simulink model "LQR_2_QuadrotorModel"  (R2023b)
settings: Solver=VariableStepAuto  StartTime=0.0  StopTime=time_model  RelTol=1e-3
values from neighbouring files (symbols this model uses):
  A_flap = [c_a, c_b, 0 ... (first row only)    [LQR_calculate.m]    (also in LQR_feedback.m; LQR_linearized_test.m; MPC_test.m; MPC_test_1.m)
  A_ind = [c_d, 0, 0 ... (first row only)    [LQR_calculate.m]    (also in LQR_feedback.m; LQR_linearized_test.m; MPC_test.m; MPC_test_1.m)
  C_drag = 0    [LQR_calculate.m]    (also in LQR_feedback.m = C_drag_arr(i); LQR_linearized_test.m = C_drag_arr(i); MPC_test.m = C_drag_arr(i); MPC_test_1.m = C_drag_arr(i))
  demp = 0    [LQR_feedback.m]    (also in LQR_linearized_test.m; MPC_params.m; MPC_test_1.m; initQuadrotorData.m)
  forward_1 = 20    [LQR_feedback.m]    (also in LQR_linearized_test.m; MPC_test_1.m)
  forward_2 = 20    [LQR_feedback.m]    (also in LQR_linearized_test.m; MPC_test_1.m)
  g = 9.81    [LQR_calculate.m]    (also in LQR_feedback.m = 9.8; LQR_linearized_test.m = 9.8; LQR_testing_gpt.m; MPC_params.m = 9.8)
  Ix = m/3*a^2/12+2*0.045*l^2    (= 0.00211347222222)    [LQR_calculate.m]    (also in LQR_feedback.m; LQR_linearized_test.m; LQR_testing_gpt.m = 0.0081; MPC_params.m)
  Iy = m/3*a^2/12+4*0.045*l^2    (= 0.00413847222222)    [LQR_calculate.m]    (also in LQR_feedback.m = 0.00211347222222; LQR_linearized_test.m = 0.00211347222222; LQR_testing_gpt.m = 0.0081; MPC_params.m = 0.00211347222222)
  Iz = m/3*a^2/4+2*0.045*l^2    (= 0.00229041666667)    [LQR_calculate.m]    (also in LQR_feedback.m = 0.00431541666667; LQR_linearized_test.m = 0.00431541666667; LQR_testing_gpt.m = 0.0142; MPC_params.m = 0.00431541666667)
  J = 2.5*10^(-6)    (= 2.5e-06)    [LQR_calculate.m]    (also in LQR_feedback.m; LQR_linearized_test.m; MPC_params.m; MPC_test.m)
  K = Y * inv(P)    [LQR_calculate.m]    (also in LQR_feedback.m = [Kx;Ky;Kz;Kphi;Ktheta;-Kpsi])
  Ke = ke    (= 0.0073)    [LQR_calculate.m]    (also in LQR_feedback.m = 0.00734; LQR_linearized_test.m = 0.00734; MPC_params.m = 0.00734; MPC_test.m)
  kf = ks*r^2*airDensity*Sblade/2    (= 1.57565625e-05)    [LQR_calculate.m]    (also in LQR_feedback.m; LQR_linearized_test.m; MPC_params.m; MPC_test.m)
  Km = kt    (= 0.0073)    [LQR_calculate.m]    (also in LQR_feedback.m = 0.00734; LQR_linearized_test.m = 0.00734; MPC_params.m = 0.00734; MPC_test.m)
  kv = 1300    [LQR_feedback.m]    (also in LQR_linearized_test.m; MPC_test_1.m; initQuadrotorData.m)
  L = La    (= 5e-05)    [LQR_calculate.m]    (also in LQR_feedback.m = 0.0001; LQR_linearized_test.m = 0.0001; MPC_params.m = 0.0001; MPC_test.m)
  l = 0.15    [LQR_calculate.m]    (also in LQR_feedback.m; LQR_linearized_test.m; MPC_params.m; MPC_test.m)
  m = size(B, 2)    [LQR_calculate.m]    (also in LQR_feedback.m = 0.65; LQR_linearized_test.m = 0.65; LQR_testing_gpt.m = 1; MPC_params.m = 0.65)
  maxU = 16    [LQR_calculate.m]    (also in LQR_feedback.m; LQR_linearized_test.m; MPC_params.m; MPC_test.m = 11)
  Mode = 3    [LQR_feedback.m]    (also in LQR_linearized_test.m; MPC_test_1.m = 1)
  phi0 = 0    [LQR_feedback.m]    (also in LQR_linearized_test.m; MPC_test_1.m)
  psi0 = pi/2    (= 1.57079632679)    [LQR_feedback.m]    (also in LQR_linearized_test.m; MPC_test_1.m = 0)
  R = eye(4)    [LQR_calculate.m]    (also in LQR_feedback.m = 0.058; LQR_linearized_test.m = 0.058; LQR_testing_gpt.m = diag([0.1, 10, 100, 10]); MPC_params.m = 0.058)
  rho = 1.225    [LQR_calculate.m]    (also in LQR_feedback.m; LQR_linearized_test.m; MPC_params.m; MPC_test.m)
  S = l*c*4+a*b    (= 0.0169)    [LQR_calculate.m]    (also in LQR_feedback.m; LQR_linearized_test.m; MPC_params.m; MPC_test.m)
  theta0 = 0    [LQR_feedback.m]    (also in LQR_linearized_test.m; MPC_test_1.m)
  total_time = 60    [LQR_feedback.m]    (also in LQR_linearized_test.m; MPC_test_1.m)
  up_down = 5    [LQR_feedback.m]    (also in LQR_linearized_test.m; MPC_test_1.m)
  x0 = 0    [LQR_feedback.m]    (also in LQR_linearized_test.m; MPC_test_1.m; init_nmpc.m = zeros(nx,1))
  y0 = 0    [LQR_feedback.m]    (also in LQR_linearized_test.m; MPC_test_1.m)
  z0 = 0    [LQR_feedback.m]    (also in LQR_linearized_test.m; MPC_test_1.m)
libraries: sharedtransform x1
settings Model: Creator=Degra  LastModifiedBy=Degra

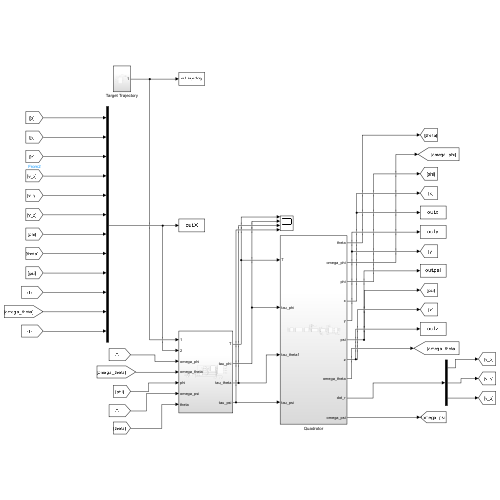
[thumbnail: Simulink's stored preview of the top-level diagram]
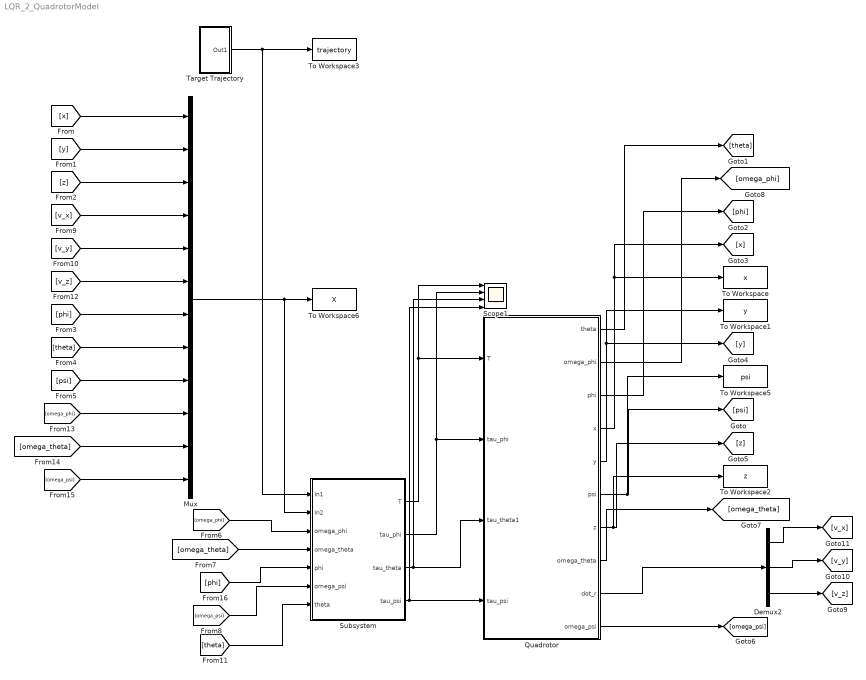
== system LQR_2_QuadrotorModel ==
  Demux2 : Demux  Outputs=3
  Mux : Mux  Inputs=12
  Quadrotor : Subsystem
  Scope1 : Scope  NumInputPorts=4
  Subsystem : Subsystem
  Target Trajectory : Subsystem
  To Workspace : ToWorkspace  VariableName=x  SaveFormat=Timeseries  SampleTime=-1
  To Workspace1 : ToWorkspace  VariableName=y  SaveFormat=Timeseries  SampleTime=-1
  To Workspace2 : ToWorkspace  VariableName=z  SaveFormat=Timeseries  SampleTime=-1
  To Workspace3 : ToWorkspace  VariableName=trajectory  SaveFormat=Timeseries  SampleTime=-1
  To Workspace5 : ToWorkspace  VariableName=psi  SaveFormat=Timeseries  SampleTime=-1
  To Workspace6 : ToWorkspace  VariableName=X  SaveFormat=Timeseries  SampleTime=-1
  wires:
  [x] -> Mux/1
  Demux2/3 -> [v_z]
  Demux2/2 -> [v_y]
  [phi] -> Subsystem/5(phi)
  [omega_psi] -> Mux/12
  [y] -> Mux/2
  [z] -> Mux/3
  [phi] -> Mux/7
  [theta] -> Subsystem/7(theta)
  [v_y] -> Mux/5
  [omega_psi] -> Subsystem/6(omega_psi)
  [v_x] -> Mux/4
  Demux2/1 -> [v_x]
  Quadrotor/5(y) -> To Workspace1/1, [y]
  Quadrotor/4(x) -> [x], To Workspace/1
  [omega_theta] -> Mux/11
  [v_z] -> Mux/6
  [psi] -> Mux/9
  [theta] -> Mux/8
  [omega_phi] -> Mux/10
  Target Trajectory/1(Out1) -> To Workspace3/1, Subsystem/1(In1)
  Mux/1 -> Subsystem/2(In2), To Workspace6/1
  Quadrotor/10(omega_psi) -> [omega_psi]
  Quadrotor/9(dot_r) -> Demux2/1
  [omega_theta] -> Subsystem/4(omega_theta)
  [omega_phi] -> Subsystem/3(omega_phi)
  Subsystem/4(tau_psi) -> Scope1/4, Quadrotor/4(tau_psi)
  Subsystem/3(tau_theta) -> Quadrotor/3(tau_theta1), Scope1/3
  Subsystem/2(tau_phi) -> Quadrotor/2(tau_phi), Scope1/2
  Subsystem/1(T) -> Scope1/1, Quadrotor/1(T)
  Quadrotor/3(phi) -> [phi]
  Quadrotor/2(omega_phi) -> [omega_phi]
  Quadrotor/1(theta) -> [theta]
  Quadrotor/8(omega_theta) -> [omega_theta]
  Quadrotor/7(z) -> To Workspace2/1, [z]
  Quadrotor/6(psi) -> [psi], To Workspace5/1

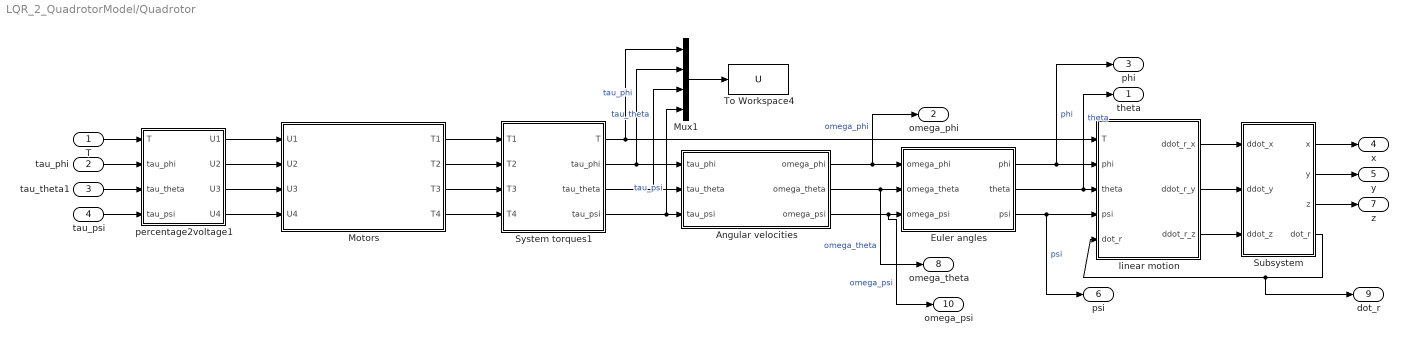
== system LQR_2_QuadrotorModel/Quadrotor ==
  T : Inport
  tau_phi : Inport  Port=2
  tau_theta1 : Inport  Port=3
  tau_psi : Inport  Port=4
  Angular velocities : Subsystem
  Euler angles : Subsystem
  Motors : Subsystem
  Mux1 : Mux
  Subsystem : Subsystem
  System torques1 : Subsystem
  To Workspace4 : ToWorkspace  VariableName=U  SaveFormat=Timeseries  SampleTime=-1
  linear motion : Subsystem
  percentage2voltage1 : Subsystem
  theta : Outport
  omega_phi : Outport  Port=2
  phi : Outport  Port=3
  x : Outport  Port=4
  y : Outport  Port=5
  psi : Outport  Port=6
  z : Outport  Port=7
  omega_theta : Outport  Port=8
  dot_r : Outport  Port=9
  omega_psi : Outport  Port=10
  wires:
  Angular velocities/1(omega_phi) -> Euler angles/1(omega_phi), omega_phi/1  "omega_phi"
  linear motion/2(ddot_r_y) -> Subsystem/2(ddot_y)
  Subsystem/4(dot_r) -> linear motion/5(dot_r), dot_r/1
  Angular velocities/2(omega_theta) -> Euler angles/2(omega_theta), omega_theta/1  "omega_theta"
  percentage2voltage1/4(U4) -> Motors/4(U4)
  tau_psi/1 -> percentage2voltage1/4(tau_psi)
  Euler angles/1(phi) -> linear motion/2(phi), phi/1  "phi"
  Euler angles/2(theta) -> linear motion/3(theta), theta/1  "theta"
  T/1 -> percentage2voltage1/1(T)
  System torques1/3(tau_theta) -> Mux1/3, Angular velocities/2(tau_theta)  "tau_theta"
  linear motion/3(ddot_r_z) -> Subsystem/3(ddot_z)
  linear motion/1(ddot_r_x) -> Subsystem/1(ddot_x)
  Motors/3(T3) -> System torques1/3(T3)
  tau_phi/1 -> percentage2voltage1/2(tau_phi)
  Euler angles/3(psi) -> linear motion/4(psi), psi/1  "psi"
  tau_theta1/1 -> percentage2voltage1/3(tau_theta)
  Motors/2(T2) -> System torques1/2(T2)
  Subsystem/3(z) -> z/1
  Motors/1(T1) -> System torques1/1(T1)
  Subsystem/1(x) -> x/1
  Motors/4(T4) -> System torques1/4(T4)
  Angular velocities/3(omega_psi) -> omega_psi/1, Euler angles/3(omega_psi)  "omega_psi"
  percentage2voltage1/3(U3) -> Motors/3(U3)
  percentage2voltage1/2(U2) -> Motors/2(U2)
  percentage2voltage1/1(U1) -> Motors/1(U1)
  System torques1/2(tau_phi) -> Mux1/2, Angular velocities/1(tau_phi)  "tau_phi"
  Subsystem/2(y) -> y/1
  System torques1/4(tau_psi) -> Mux1/4, Angular velocities/3(tau_psi)  "tau_psi"
  Mux1/1 -> To Workspace4/1
  System torques1/1(T) -> Mux1/1, linear motion/1(T)

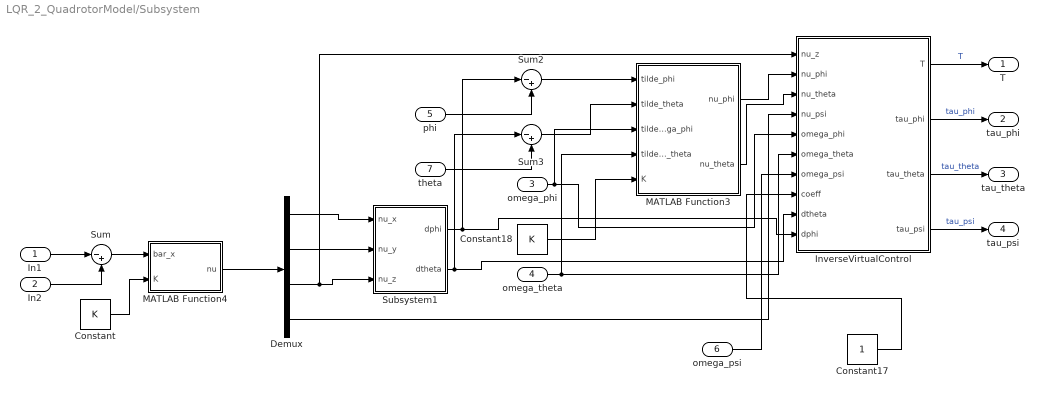
== system LQR_2_QuadrotorModel/Subsystem ==
  In1 : Inport
  In2 : Inport  Port=2
  omega_phi : Inport  Port=3
  omega_theta : Inport  Port=4
  phi : Inport  Port=5
  omega_psi : Inport  Port=6
  theta : Inport  Port=7
  Constant : Constant  Value=K
  Constant17 : Constant
  Constant18 : Constant  Value=K
  Demux : Demux
  InverseVirtualControl : Subsystem
  MATLAB Function3 : MATLAB Function  TreatAsAtomicUnit=on
  MATLAB Function4 : MATLAB Function  TreatAsAtomicUnit=on
  Subsystem1 : Subsystem
  Sum : Sum  Inputs=|-+
  Sum2 : Sum  Inputs=|-+
  Sum3 : Sum  Inputs=|-+
  T : Outport
  tau_phi : Outport  Port=2
  tau_theta : Outport  Port=3
  tau_psi : Outport  Port=4
  wires:
  In1/1 -> Sum/1
  Demux/1 -> Subsystem1/1(nu_x)
  omega_phi/1 -> InverseVirtualControl/5(omega_phi), MATLAB Function3/3(tilde_omega_phi)
  In2/1 -> Sum/2
  MATLAB Function4/1(nu) -> Demux/1
  Sum/1 -> MATLAB Function4/1(bar_x)
  Constant/1 -> MATLAB Function4/2(K)
  Demux/2 -> Subsystem1/2(nu_y)
  Subsystem1/2(dtheta) -> Sum3/1, InverseVirtualControl/9(dtheta)
  Demux/4 -> InverseVirtualControl/4(nu_psi)
  Demux/3 -> InverseVirtualControl/1(nu_z), Subsystem1/3(nu_z)
  omega_theta/1 -> InverseVirtualControl/6(omega_theta), MATLAB Function3/4(tilde_omega_theta)
  Sum2/1 -> MATLAB Function3/1(tilde_phi)
  phi/1 -> Sum2/2
  omega_psi/1 -> InverseVirtualControl/7(omega_psi)
  theta/1 -> Sum3/2
  Subsystem1/1(dphi) -> InverseVirtualControl/10(dphi), Sum2/1
  Sum3/1 -> MATLAB Function3/2(tilde_theta)
  Constant17/1 -> InverseVirtualControl/8(coeff)
  Constant18/1 -> MATLAB Function3/5(K)
  MATLAB Function3/2(nu_theta) -> InverseVirtualControl/3(nu_theta)
  MATLAB Function3/1(nu_phi) -> InverseVirtualControl/2(nu_phi)
  InverseVirtualControl/2(tau_phi) -> tau_phi/1  "tau_phi"
  InverseVirtualControl/1(T) -> T/1  "T"
  InverseVirtualControl/4(tau_psi) -> tau_psi/1  "tau_psi"
  InverseVirtualControl/3(tau_theta) -> tau_theta/1  "tau_theta"

== system LQR_2_QuadrotorModel/Target Trajectory ==
  Clock : Clock
  Clock2 : Clock
  Constant1 : Constant  Value=Mode
  Constant13 : Constant  Value=forward_2
  Constant14 : Constant  Value=total_time
  Constant15 : Constant  Value=up_down
  Constant16 : Constant  Value=forward_1
  MATLAB Function : MATLAB Function  TreatAsAtomicUnit=on
  MATLAB Function1 : MATLAB Function  TreatAsAtomicUnit=on
  Multiport Switch : MultiPortSwitch  Inputs=2  SaturateOnIntegerOverflow=off  InputSameDT=off
  Out1 : Outport
  wires:
  Constant1/1 -> Multiport Switch/1
  Clock/1 -> MATLAB Function1/1(t)
  Constant13/1 -> MATLAB Function/2(forward_20)
  Clock2/1 -> MATLAB Function/1(t)
  MATLAB Function/1(x_ref) -> Multiport Switch/3
  Constant14/1 -> MATLAB Function/5(total_time)
  Multiport Switch/1 -> Out1/1
  Constant16/1 -> MATLAB Function/3(forward_10)
  MATLAB Function1/1(x_ref) -> Multiport Switch/2
  Constant15/1 -> MATLAB Function/4(up_down)

== system LQR_2_QuadrotorModel/Quadrotor/Angular velocities ==
  tau_phi : Inport
  tau_theta : Inport  Port=2
  tau_psi : Inport  Port=3
  Subsystem1 : Subsystem
  Subsystem2 : Subsystem
  Subsystem3 : Subsystem
  omega_phi : Outport
  omega_theta : Outport  Port=2
  omega_psi : Outport  Port=3
  wires:
  Subsystem2/1(omega_theta) -> omega_theta/1, Subsystem1/2(omega_theta), Subsystem3/3(omega_theta)  "omega_theta"
  tau_theta/1 -> Subsystem2/1(tau_theta)
  Subsystem1/1(omega_phi) -> omega_phi/1, Subsystem3/2(omega_phi), Subsystem2/2(omega_phi)  "omega_phi"
  Subsystem3/1(omega_psi) -> omega_psi/1, Subsystem2/3(omega_psi), Subsystem1/3(omega_psi)  "omega_psi"
  tau_phi/1 -> Subsystem1/1(tau_phi)
  tau_psi/1 -> Subsystem3/1(tau_psi)

== system LQR_2_QuadrotorModel/Quadrotor/Euler angles ==
  omega_phi : Inport
  omega_theta : Inport  Port=2
  omega_psi : Inport  Port=3
  Subsystem1 : Subsystem
  Subsystem2 : Subsystem
  Subsystem3 : Subsystem
  phi : Outport
  theta : Outport  Port=2
  psi : Outport  Port=3
  wires:
  Subsystem2/1(theta) -> theta/1, Subsystem1/2(theta), Subsystem3/4(theta)  "theta"
  Subsystem1/1(phi) -> phi/1, Subsystem3/1(phi), Subsystem2/1(phi)  "phi"
  omega_theta/1 -> Subsystem3/2(omega_theta), Subsystem1/3(omega_theta), Subsystem2/2(omega_theta)
  omega_psi/1 -> Subsystem2/3(omega_psi), Subsystem3/3(omega_psi), Subsystem1/4(omega_psi)
  omega_phi/1 -> Subsystem1/1(omega_phi)
  Subsystem3/1(psi) -> psi/1  "psi"

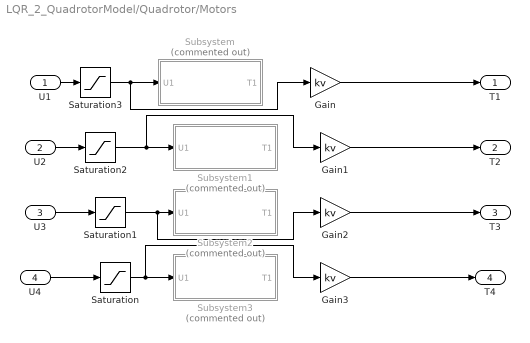
== system LQR_2_QuadrotorModel/Quadrotor/Motors ==
  U1 : Inport
  U2 : Inport  Port=2
  U3 : Inport  Port=3
  U4 : Inport  Port=4
  Gain{,1..3} (4 alike) : Gain  Gain=kv
  Saturation{,1..3} (4 alike) : Saturate  UpperLimit=maxU  LowerLimit=-maxU
  Subsystem : Subsystem  Commented=on
  Subsystem1 : Subsystem  Commented=on
  Subsystem2 : Subsystem  Commented=on
  Subsystem3 : Subsystem  Commented=on
  T1 : Outport
  T2 : Outport  Port=2
  T3 : Outport  Port=3
  T4 : Outport  Port=4
  wires:
  U4/1 -> Saturation/1
  U1/1 -> Saturation3/1
  U3/1 -> Saturation1/1
  U2/1 -> Saturation2/1
  Gain/1 -> T1/1
  Gain1/1 -> T2/1
  Gain2/1 -> T3/1
  Gain3/1 -> T4/1
  Saturation/1 -> Gain3/1, Subsystem3/1(U1)
  Saturation1/1 -> Gain2/1, Subsystem2/1(U1)
  Saturation2/1 -> Gain1/1, Subsystem1/1(U1)
  Saturation3/1 -> Gain/1, Subsystem/1(U1)

== system LQR_2_QuadrotorModel/Quadrotor/Subsystem ==
  ddot_x : Inport
  ddot_y : Inport  Port=2
  ddot_z : Inport  Port=3
  Integrator10 : Integrator  InitialCondition=z0
  Integrator11 : Integrator
  Integrator6 : Integrator  InitialCondition=x0
  Integrator7 : Integrator
  Integrator8 : Integrator  InitialCondition=y0
  Integrator9 : Integrator
  Mux : Mux  Inputs=3
  x : Outport
  y : Outport  Port=2
  z : Outport  Port=3
  dot_r : Outport  Port=4
  wires:
  Integrator9/1 -> Mux/2, Integrator8/1
  Integrator7/1 -> Mux/1, Integrator6/1
  Integrator10/1 -> z/1  "z"
  Integrator11/1 -> Mux/3, Integrator10/1
  Integrator8/1 -> y/1  "y"
  ddot_x/1 -> Integrator7/1
  Mux/1 -> dot_r/1  "dot_r"
  Integrator6/1 -> x/1  "x"
  ddot_y/1 -> Integrator9/1
  ddot_z/1 -> Integrator11/1

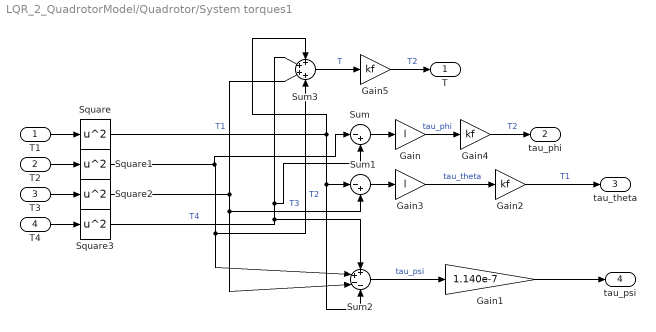
== system LQR_2_QuadrotorModel/Quadrotor/System torques1 ==
  T1 : Inport
  T2 : Inport  Port=2
  T3 : Inport  Port=3
  T4 : Inport  Port=4
  Gain : Gain  Gain=l
  Gain1 : Gain  Gain=1.140e-7
  Gain2 : Gain  Gain=kf
  Gain3 : Gain  Gain=l
  Gain4 : Gain  Gain=kf
  Gain5 : Gain  Gain=kf
  Square{,1..3} (4 alike) : Math  Operator=square
  Sum : Sum  Inputs=|-+
  Sum1 : Sum  Inputs=|-+
  Sum2 : Sum  Inputs=++--
  Sum3 : Sum  Inputs=++++
  T : Outport
  tau_phi : Outport  Port=2
  tau_theta : Outport  Port=3
  tau_psi : Outport  Port=4
  wires:
  T3/1 -> Square2/1
  T4/1 -> Square3/1
  Sum2/1 -> Gain1/1  "tau_psi"
  T1/1 -> Square/1
  Sum/1 -> Gain/1
  Sum1/1 -> Gain3/1
  Sum3/1 -> Gain5/1  "T"
  T2/1 -> Square1/1
  Gain3/1 -> Gain2/1  "tau_theta"
  Gain/1 -> Gain4/1  "tau_phi"
  Gain1/1 -> tau_psi/1
  Square/1 -> Sum1/1, Sum2/4, Sum3/1  "T1"
  Square1/1 -> Sum/1, Sum2/2, Sum3/4  "T2"
  Square2/1 -> Sum1/2, Sum2/3, Sum3/3  "T3"
  Square3/1 -> Sum/2, Sum3/2, Sum2/1  "T4"
  Gain4/1 -> tau_phi/1  "T2"
  Gain2/1 -> tau_theta/1  "T1"
  Gain5/1 -> T/1  "T2"

== system LQR_2_QuadrotorModel/Quadrotor/linear motion ==
  T : Inport
  phi : Inport  Port=2
  theta : Inport  Port=3
  psi : Inport  Port=4
  dot_r : Inport  Port=5
  Subsystem : Subsystem
  Subsystem1 : Subsystem
  Subsystem2 : Subsystem
  Subsystem3 : Subsystem
  ddot_r_x : Outport
  ddot_r_y : Outport  Port=2
  ddot_r_z : Outport  Port=3
  wires:
  T/1 -> Subsystem/1(T), Subsystem2/2(T), Subsystem3/1(T), Subsystem1/1(T)
  theta/1 -> Subsystem/2(theta), Subsystem2/3(theta), Subsystem3/4(theta), Subsystem1/3(theta)
  phi/1 -> Subsystem/3(phi), Subsystem2/4(phi), Subsystem3/2(phi), Subsystem1/2(phi)
  Subsystem1/3((F_ind+F_flap+F_drag)_z) -> Subsystem/4((F_ind+F_flap+F_drag)_z)
  psi/1 -> Subsystem3/5(psi), Subsystem2/1(psi), Subsystem1/4(psi)
  dot_r/1 -> Subsystem1/5(dot_r)
  Subsystem1/2((F_ind+F_flap+F_drag)_y) -> Subsystem2/5((F_ind+F_flap+F_drag)_y)
  Subsystem1/1((F_ind+F_flap+F_drag)_x) -> Subsystem3/3((F_ind+F_flap+F_drag)_x)
  Subsystem3/1(ddot_r_x) -> ddot_r_x/1  "ddot_r_x"
  Subsystem2/1(ddot_r_y) -> ddot_r_y/1  "ddot_r_y"
  Subsystem/1(ddot_r_z) -> ddot_r_z/1  "ddot_r_z"

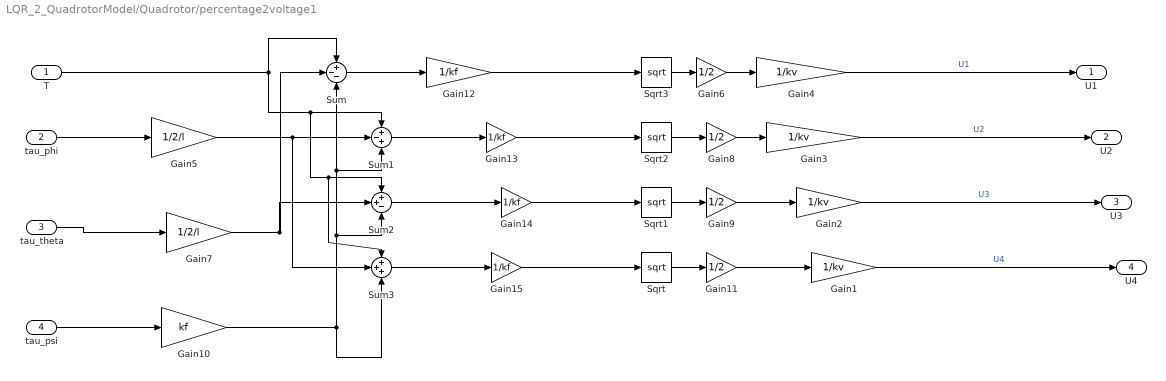
== system LQR_2_QuadrotorModel/Quadrotor/percentage2voltage1 ==
  T : Inport
  tau_phi : Inport  Port=2
  tau_theta : Inport  Port=3
  tau_psi : Inport  Port=4
  Gain{1..4} (4 alike) : Gain  Gain=1/kv
  Gain10 : Gain  Gain=kf
  Gain{6,8..9,11} (4 alike) : Gain  Gain=1/2
  Gain{12..15} (4 alike) : Gain  Gain=1/kf
  Gain5 : Gain  Gain=1/2/l
  Gain7 : Gain  Gain=1/2/l
  Sqrt{,1..3} (4 alike) : Sqrt
  Sum : Sum  Inputs=+--
  Sum1 : Sum  Inputs=+-+
  Sum2 : Sum  Inputs=++-
  Sum3 : Sum  Inputs=+++
  U1 : Outport
  U2 : Outport  Port=2
  U3 : Outport  Port=3
  U4 : Outport  Port=4
  wires:
  Gain2/1 -> U3/1  "U3"
  Gain4/1 -> U1/1  "U1"
  Gain3/1 -> U2/1  "U2"
  Gain1/1 -> U4/1  "U4"
  Sum3/1 -> Gain15/1
  Sum2/1 -> Gain14/1
  tau_phi/1 -> Gain5/1
  tau_theta/1 -> Gain7/1
  tau_psi/1 -> Gain10/1
  Gain10/1 -> Sum3/3, Sum1/3, Sum/3, Sum2/3
  Sqrt/1 -> Gain11/1
  Sqrt1/1 -> Gain9/1
  Sqrt2/1 -> Gain8/1
  Sqrt3/1 -> Gain6/1
  Gain6/1 -> Gain4/1
  Gain8/1 -> Gain3/1
  Gain9/1 -> Gain2/1
  Gain11/1 -> Gain1/1
  Sum/1 -> Gain12/1
  Sum1/1 -> Gain13/1
  Gain14/1 -> Sqrt1/1
  Gain15/1 -> Sqrt/1
  Gain5/1 -> Sum3/2, Sum1/2
  Gain7/1 -> Sum2/2, Sum/2
  T/1 -> Sum3/1, Sum2/1, Sum1/1, Sum/1
  Gain12/1 -> Sqrt3/1
  Gain13/1 -> Sqrt2/1

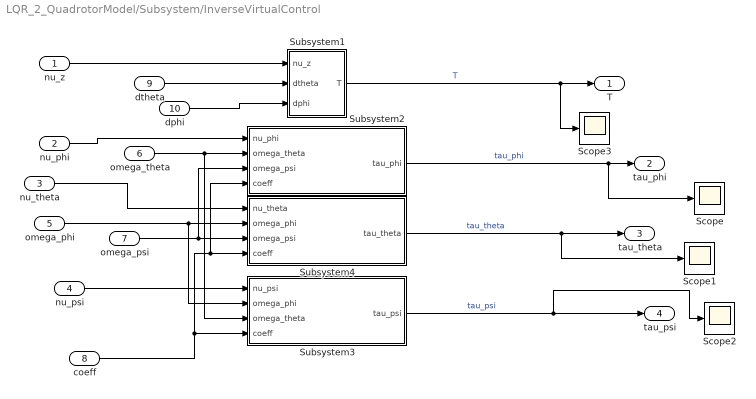
== system LQR_2_QuadrotorModel/Subsystem/InverseVirtualControl ==
  nu_z : Inport
  nu_phi : Inport  Port=2
  nu_theta : Inport  Port=3
  nu_psi : Inport  Port=4
  omega_phi : Inport  Port=5
  omega_theta : Inport  Port=6
  omega_psi : Inport  Port=7
  coeff : Inport  Port=8
  dtheta : Inport  Port=9
  dphi : Inport  Port=10
  Scope{,1..3} (4 alike) : Scope
  Subsystem1 : Subsystem
  Subsystem2 : Subsystem
  Subsystem3 : Subsystem
  Subsystem4 : Subsystem
  T : Outport
  tau_phi : Outport  Port=2
  tau_theta : Outport  Port=3
  tau_psi : Outport  Port=4
  wires:
  nu_psi/1 -> Subsystem3/1(nu_psi)
  omega_psi/1 -> Subsystem2/3(omega_psi), Subsystem4/3(omega_psi)
  omega_theta/1 -> Subsystem3/3(omega_theta), Subsystem2/2(omega_theta)
  nu_phi/1 -> Subsystem2/1(nu_phi)
  omega_phi/1 -> Subsystem3/2(omega_phi), Subsystem4/2(omega_phi)
  coeff/1 -> Subsystem2/4(coeff), Subsystem4/4(coeff), Subsystem3/4(coeff)
  nu_z/1 -> Subsystem1/1(nu_z)
  Subsystem2/1(tau_phi) -> Scope/1, tau_phi/1  "tau_phi"
  nu_theta/1 -> Subsystem4/1(nu_theta)
  Subsystem1/1(T) -> Scope3/1, T/1  "T"
  Subsystem4/1(tau_theta) -> Scope1/1, tau_theta/1  "tau_theta"
  Subsystem3/1(tau_psi) -> Scope2/1, tau_psi/1  "tau_psi"
  dtheta/1 -> Subsystem1/2(dtheta)
  dphi/1 -> Subsystem1/3(dphi)

== system LQR_2_QuadrotorModel/Subsystem/Subsystem1 ==
  nu_x : Inport
  nu_y : Inport  Port=2
  nu_z : Inport  Port=3
  Atan : Trigonometry  Operator=atan2
  Atan1 : Trigonometry  Operator=atan2
  Constant18 : Constant  Value=g
  Constant19 : Constant  Value=g
  Sum3 : Sum  Inputs=|++
  Sum4 : Sum  Inputs=|++
  dphi : Outport
  dtheta : Outport  Port=2
  wires:
  Sum4/1 -> Atan1/2
  nu_x/1 -> Atan/1
  Sum3/1 -> Atan/2
  nu_y/1 -> Atan1/1
  Constant19/1 -> Sum4/2
  Constant18/1 -> Sum3/2
  nu_z/1 -> Sum3/1, Sum4/1
  Atan1/1 -> dtheta/1
  Atan/1 -> dphi/1

== system LQR_2_QuadrotorModel/Quadrotor/Angular velocities/Subsystem1 ==
  tau_phi : Inport
  omega_theta : Inport  Port=2
  omega_psi : Inport  Port=3
  Gain : Gain  Gain=Iy-Iz
  Gain1 : Gain  Gain=1/Ix
  Integrator12 : Integrator
  Product : Product
  Sum : Sum  Inputs=|++
  omega_phi : Outport
  wires:
  Gain/1 -> Sum/2
  omega_theta/1 -> Product/1
  Product/1 -> Gain/1
  Sum/1 -> Gain1/1  "dot_omega_phi"
  tau_phi/1 -> Sum/1
  omega_psi/1 -> Product/2
  Gain1/1 -> Integrator12/1
  Integrator12/1 -> omega_phi/1  "omega_phi"

== system LQR_2_QuadrotorModel/Quadrotor/Angular velocities/Subsystem2 ==
  tau_theta : Inport
  omega_phi : Inport  Port=2
  omega_psi : Inport  Port=3
  Gain : Gain  Gain=Iz-Ix
  Gain1 : Gain  Gain=1/Iy
  Integrator12 : Integrator
  Product : Product
  Sum : Sum  Inputs=|++
  omega_theta : Outport
  wires:
  Gain/1 -> Sum/2
  Sum/1 -> Gain1/1  "omega_theta"
  omega_phi/1 -> Product/1
  Product/1 -> Gain/1
  tau_theta/1 -> Sum/1
  omega_psi/1 -> Product/2
  Gain1/1 -> Integrator12/1
  Integrator12/1 -> omega_theta/1  "omega_theta"

== system LQR_2_QuadrotorModel/Quadrotor/Angular velocities/Subsystem3 ==
  tau_psi : Inport
  omega_phi : Inport  Port=2
  omega_theta : Inport  Port=3
  Gain : Gain  Gain=Ix-Iy
  Gain1 : Gain  Gain=1/Iz
  Integrator12 : Integrator
  Product : Product
  Sum : Sum  Inputs=|++
  omega_psi : Outport
  wires:
  Gain/1 -> Sum/2
  omega_phi/1 -> Product/1
  Product/1 -> Gain/1
  Sum/1 -> Gain1/1  "dot_omega_psi"
  tau_psi/1 -> Sum/1
  omega_theta/1 -> Product/2
  Gain1/1 -> Integrator12/1
  Integrator12/1 -> omega_psi/1  "omega_psi"

== system LQR_2_QuadrotorModel/Quadrotor/Euler angles/Subsystem1 ==
  omega_phi : Inport
  theta : Inport  Port=2
  omega_theta : Inport  Port=3
  omega_psi : Inport  Port=4
  Integrator : Integrator  InitialCondition=phi0
  Product : Product
  Product1 : Product
  Product2 : Product
  Sum : Sum  Inputs=|++
  Sum1 : Sum  Inputs=|++
  Tan : Trigonometry  Operator=tan
  Tan1 : Trigonometry
  Tan2 : Trigonometry  Operator=cos
  phi : Outport
  wires:
  Product2/1 -> Sum1/2
  Tan1/1 -> Product1/2
  Sum/1 -> Integrator/1
  Sum1/1 -> Product/2
  Tan/1 -> Product/1
  Tan2/1 -> Product2/2
  Product1/1 -> Sum1/1
  omega_psi/1 -> Product2/1
  omega_theta/1 -> Product1/1
  Integrator/1 -> Tan1/1, Tan2/1, phi/1  "phi"
  theta/1 -> Tan/1
  omega_phi/1 -> Sum/1
  Product/1 -> Sum/2

== system LQR_2_QuadrotorModel/Quadrotor/Euler angles/Subsystem2 ==
  phi : Inport
  omega_theta : Inport  Port=2
  omega_psi : Inport  Port=3
  Integrator : Integrator  InitialCondition=theta0
  Product1 : Product
  Product2 : Product
  Sum1 : Sum  Inputs=|+-
  Tan1 : Trigonometry  Operator=cos
  Tan2 : Trigonometry
  theta : Outport
  wires:
  Product2/1 -> Sum1/2
  Tan1/1 -> Product1/2
  Tan2/1 -> Product2/2
  Product1/1 -> Sum1/1
  omega_psi/1 -> Product2/1
  Integrator/1 -> theta/1  "theta"
  phi/1 -> Tan2/1, Tan1/1
  omega_theta/1 -> Product1/1
  Sum1/1 -> Integrator/1

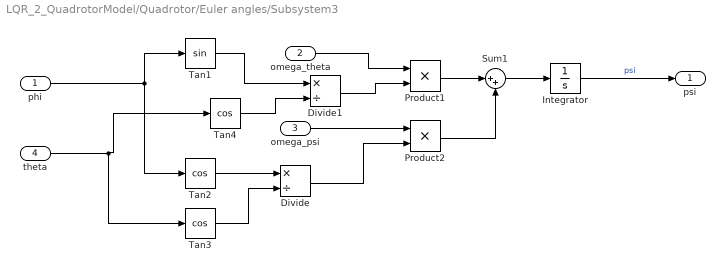
== system LQR_2_QuadrotorModel/Quadrotor/Euler angles/Subsystem3 ==
  phi : Inport
  omega_theta : Inport  Port=2
  omega_psi : Inport  Port=3
  theta : Inport  Port=4
  Divide : Product  Inputs=*/
  Divide1 : Product  Inputs=*/
  Integrator : Integrator  InitialCondition=psi0
  Product1 : Product
  Product2 : Product
  Sum1 : Sum  Inputs=|++
  Tan1 : Trigonometry
  Tan2 : Trigonometry  Operator=cos
  Tan3 : Trigonometry  Operator=cos
  Tan4 : Trigonometry  Operator=cos
  psi : Outport
  wires:
  Product2/1 -> Sum1/2
  Product1/1 -> Sum1/1
  omega_psi/1 -> Product2/1
  Integrator/1 -> psi/1  "psi"
  phi/1 -> Tan1/1, Tan2/1
  theta/1 -> Tan4/1, Tan3/1
  Divide/1 -> Product2/2
  Tan2/1 -> Divide/1
  Tan3/1 -> Divide/2
  Divide1/1 -> Product1/2
  Tan1/1 -> Divide1/1
  Tan4/1 -> Divide1/2
  omega_theta/1 -> Product1/1
  Sum1/1 -> Integrator/1

== system LQR_2_QuadrotorModel/Quadrotor/Motors/Subsystem ==
  U1 : Inport
  Add : Sum  Inputs=+--
  Add1 : Sum  Inputs=+-
  Gain : Gain  Gain=demp
  Gain1 : Gain  Gain=Km
  Gain2 : Gain  Gain=1/L
  Gain3 : Gain  Gain=Ke
  Gain5 : Gain  Gain=R
  Gain6 : Gain  Gain=1/J
  Integrator : Integrator
  Integrator1 : Integrator
  T1 : Outport
  wires:
  Gain2/1 -> Integrator/1
  Add/1 -> Gain2/1
  Integrator/1 -> Gain1/1, Gain5/1
  Gain5/1 -> Add/3
  U1/1 -> Add/1
  Gain1/1 -> Add1/1
  Add1/1 -> Gain6/1
  Integrator1/1 -> T1/1, Gain3/1, Gain/1
  Gain3/1 -> Add/2
  Gain/1 -> Add1/2
  Gain6/1 -> Integrator1/1

== system LQR_2_QuadrotorModel/Quadrotor/Motors/Subsystem1 ==
  U1 : Inport
  Add : Sum  Inputs=+--
  Add1 : Sum  Inputs=+-
  Gain : Gain  Gain=demp
  Gain1 : Gain  Gain=Km
  Gain2 : Gain  Gain=1/L
  Gain3 : Gain  Gain=Ke
  Gain5 : Gain  Gain=R
  Gain6 : Gain  Gain=1/J
  Integrator : Integrator
  Integrator1 : Integrator
  T1 : Outport
  wires:
  Gain2/1 -> Integrator/1
  Add/1 -> Gain2/1
  Integrator/1 -> Gain1/1, Gain5/1
  Gain5/1 -> Add/3
  U1/1 -> Add/1
  Gain1/1 -> Add1/1
  Add1/1 -> Gain6/1
  Integrator1/1 -> T1/1, Gain3/1, Gain/1
  Gain3/1 -> Add/2
  Gain/1 -> Add1/2
  Gain6/1 -> Integrator1/1

== system LQR_2_QuadrotorModel/Quadrotor/Motors/Subsystem2 ==
  U1 : Inport
  Add : Sum  Inputs=+--
  Add1 : Sum  Inputs=+-
  Gain : Gain  Gain=demp
  Gain1 : Gain  Gain=Km
  Gain2 : Gain  Gain=1/L
  Gain3 : Gain  Gain=Ke
  Gain5 : Gain  Gain=R
  Gain6 : Gain  Gain=1/J
  Integrator : Integrator
  Integrator1 : Integrator
  T1 : Outport
  wires:
  Gain2/1 -> Integrator/1
  Add/1 -> Gain2/1
  Integrator/1 -> Gain1/1, Gain5/1
  Gain5/1 -> Add/3
  U1/1 -> Add/1
  Gain1/1 -> Add1/1
  Add1/1 -> Gain6/1
  Integrator1/1 -> T1/1, Gain3/1, Gain/1
  Gain3/1 -> Add/2
  Gain/1 -> Add1/2
  Gain6/1 -> Integrator1/1

== system LQR_2_QuadrotorModel/Quadrotor/Motors/Subsystem3 ==
  U1 : Inport
  Add : Sum  Inputs=+--
  Add1 : Sum  Inputs=+-
  Gain : Gain  Gain=demp
  Gain1 : Gain  Gain=Km
  Gain2 : Gain  Gain=1/L
  Gain3 : Gain  Gain=Ke
  Gain5 : Gain  Gain=R
  Gain6 : Gain  Gain=1/J
  Integrator : Integrator
  Integrator1 : Integrator
  T1 : Outport
  wires:
  Gain2/1 -> Integrator/1
  Add/1 -> Gain2/1
  Integrator/1 -> Gain1/1, Gain5/1
  Gain5/1 -> Add/3
  U1/1 -> Add/1
  Gain1/1 -> Add1/1
  Add1/1 -> Gain6/1
  Integrator1/1 -> T1/1, Gain3/1, Gain/1
  Gain3/1 -> Add/2
  Gain/1 -> Add1/2
  Gain6/1 -> Integrator1/1

== system LQR_2_QuadrotorModel/Quadrotor/linear motion/Subsystem ==
  T : Inport
  theta : Inport  Port=2
  phi : Inport  Port=3
  (F_ind+F_flap+F_drag)_z : Inport  Port=4
  Constant4 : Constant  Value=m*g
  Cos4 : Trigonometry  Operator=cos
  Cos5 : Trigonometry  Operator=cos
  Gain4 : Gain  Gain=1/m
  Product2 : Product  Inputs=3
  Sum2 : Sum  Inputs=|+--
  ddot_r_z : Outport
  wires:
  Product2/1 -> Sum2/1
  phi/1 -> Cos4/1
  theta/1 -> Cos5/1
  T/1 -> Product2/1
  Cos4/1 -> Product2/2
  Constant4/1 -> Sum2/3
  Cos5/1 -> Product2/3
  (F_ind+F_flap+F_drag)_z/1 -> Sum2/2
  Sum2/1 -> Gain4/1
  Gain4/1 -> ddot_r_z/1  "ddot_r_z"

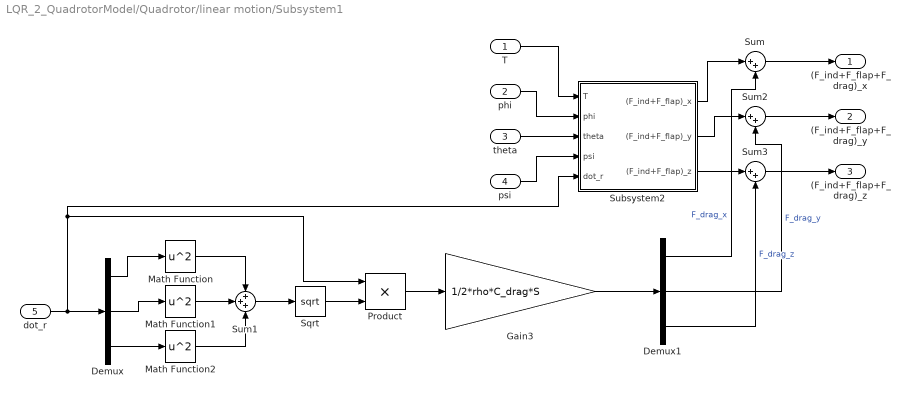
== system LQR_2_QuadrotorModel/Quadrotor/linear motion/Subsystem1 ==
  T : Inport
  phi : Inport  Port=2
  theta : Inport  Port=3
  psi : Inport  Port=4
  dot_r : Inport  Port=5
  Demux : Demux  Outputs=3
  Demux1 : Demux  Outputs=3
  Gain3 : Gain  Gain=1/2*rho*C_drag*S
  Math Function : Math  Operator=square
  Math Function1 : Math  Operator=square
  Math Function2 : Math  Operator=square
  Product : Product
  Sqrt : Sqrt
  Subsystem2 : Subsystem
  Sum : Sum  Inputs=|++
  Sum1 : Sum  Inputs=+++
  Sum2 : Sum  Inputs=|++
  Sum3 : Sum  Inputs=|++
  (F_ind+F_flap+F_drag)_x : Outport
  (F_ind+F_flap+F_drag)_y : Outport  Port=2
  (F_ind+F_flap+F_drag)_z : Outport  Port=3
  wires:
  Demux1/2 -> Sum2/2  "F_drag_y"
  dot_r/1 -> Product/1, Subsystem2/5(dot_r), Demux/1
  Math Function1/1 -> Sum1/2
  Demux/1 -> Math Function/1
  Demux/2 -> Math Function1/1
  Sum1/1 -> Sqrt/1
  Math Function/1 -> Sum1/1
  Demux/3 -> Math Function2/1
  Demux1/3 -> Sum3/2  "F_drag_z"
  Subsystem2/2((F_ind+F_flap)_y) -> Sum2/1
  Math Function2/1 -> Sum1/3
  Sqrt/1 -> Product/2
  phi/1 -> Subsystem2/2(phi)
  Product/1 -> Gain3/1
  T/1 -> Subsystem2/1(T)
  theta/1 -> Subsystem2/3(theta)
  psi/1 -> Subsystem2/4(psi)
  Gain3/1 -> Demux1/1
  Subsystem2/1((F_ind+F_flap)_x) -> Sum/1
  Subsystem2/3((F_ind+F_flap)_z) -> Sum3/1
  Demux1/1 -> Sum/2  "F_drag_x"
  Sum/1 -> (F_ind+F_flap+F_drag)_x/1
  Sum2/1 -> (F_ind+F_flap+F_drag)_y/1
  Sum3/1 -> (F_ind+F_flap+F_drag)_z/1

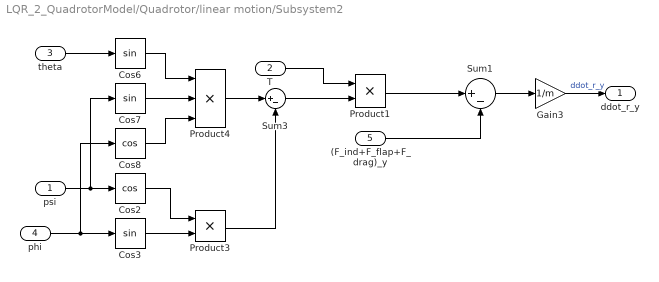
== system LQR_2_QuadrotorModel/Quadrotor/linear motion/Subsystem2 ==
  psi : Inport
  T : Inport  Port=2
  theta : Inport  Port=3
  phi : Inport  Port=4
  (F_ind+F_flap+F_drag)_y : Inport  Port=5
  Cos2 : Trigonometry  Operator=cos
  Cos3 : Trigonometry
  Cos6 : Trigonometry
  Cos7 : Trigonometry
  Cos8 : Trigonometry  Operator=cos
  Gain3 : Gain  Gain=1/m
  Product1 : Product
  Product3 : Product
  Product4 : Product  Inputs=3
  Sum1 : Sum  Inputs=|+-
  Sum3 : Sum  Inputs=|+-
  ddot_r_y : Outport
  wires:
  Cos6/1 -> Product4/1
  theta/1 -> Cos6/1
  psi/1 -> Cos7/1, Cos2/1
  Cos7/1 -> Product4/2
  Sum1/1 -> Gain3/1
  phi/1 -> Cos8/1, Cos3/1
  Cos8/1 -> Product4/3
  Cos2/1 -> Product3/1
  Cos3/1 -> Product3/2
  Product4/1 -> Sum3/1
  Product3/1 -> Sum3/2
  T/1 -> Product1/1
  Sum3/1 -> Product1/2
  Product1/1 -> Sum1/1
  (F_ind+F_flap+F_drag)_y/1 -> Sum1/2
  Gain3/1 -> ddot_r_y/1  "ddot_r_y"

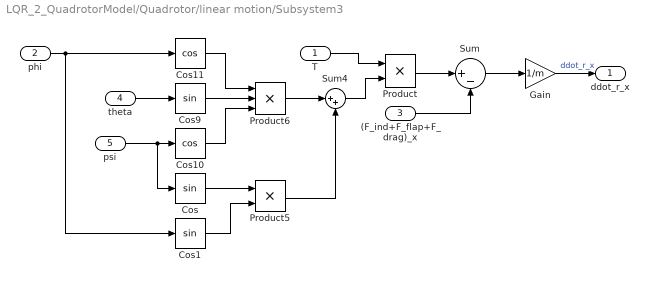
== system LQR_2_QuadrotorModel/Quadrotor/linear motion/Subsystem3 ==
  T : Inport
  phi : Inport  Port=2
  (F_ind+F_flap+F_drag)_x : Inport  Port=3
  theta : Inport  Port=4
  psi : Inport  Port=5
  Cos : Trigonometry
  Cos1 : Trigonometry
  Cos10 : Trigonometry  Operator=cos
  Cos11 : Trigonometry  Operator=cos
  Cos9 : Trigonometry
  Gain : Gain  Gain=1/m
  Product : Product
  Product5 : Product
  Product6 : Product  Inputs=3
  Sum : Sum  Inputs=|+-
  Sum4 : Sum  Inputs=|++
  ddot_r_x : Outport
  wires:
  theta/1 -> Cos9/1
  Cos/1 -> Product5/1
  psi/1 -> Cos10/1, Cos/1
  Cos11/1 -> Product6/1
  Sum/1 -> Gain/1
  (F_ind+F_flap+F_drag)_x/1 -> Sum/2
  phi/1 -> Cos11/1, Cos1/1
  Cos1/1 -> Product5/2
  Cos9/1 -> Product6/2
  Cos10/1 -> Product6/3
  Product6/1 -> Sum4/1
  Product5/1 -> Sum4/2
  T/1 -> Product/1
  Sum4/1 -> Product/2
  Product/1 -> Sum/1
  Gain/1 -> ddot_r_x/1  "ddot_r_x"

== system LQR_2_QuadrotorModel/Subsystem/InverseVirtualControl/Subsystem1 ==
  nu_z : Inport
  dtheta : Inport  Port=2
  dphi : Inport  Port=3
  Constant17 : Constant  Value=g
  Cos : Trigonometry  Operator=cos
  Cos1 : Trigonometry  Operator=cos
  Divide : Product  Inputs=*/
  Gain : Gain  Gain=m
  Product : Product
  Scope{,1..3} (4 alike) : Scope
  Sum2 : Sum  Inputs=++|
  T : Outport
  wires:
  nu_z/1 -> Sum2/1, Scope/1
  Cos/1 -> Product/1
  Constant17/1 -> Sum2/2
  Product/1 -> Scope2/1, Divide/2
  Sum2/1 -> Gain/1
  Cos1/1 -> Product/2
  Divide/1 -> Scope3/1, T/1  "T"
  Gain/1 -> Scope1/1, Divide/1
  dtheta/1 -> Cos/1
  dphi/1 -> Cos1/1

== system LQR_2_QuadrotorModel/Subsystem/InverseVirtualControl/Subsystem2 ==
  nu_phi : Inport
  omega_theta : Inport  Port=2
  omega_psi : Inport  Port=3
  coeff : Inport  Port=4
  Gain : Gain  Gain=Iy-Iz
  Gain1 : Gain  Gain=Ix
  Product : Product  Inputs=3
  Sum2 : Sum  Inputs=+-
  tau_phi : Outport
  wires:
  omega_theta/1 -> Product/1
  Gain1/1 -> Sum2/1
  nu_phi/1 -> Gain1/1
  coeff/1 -> Product/3
  Product/1 -> Gain/1
  Sum2/1 -> tau_phi/1  "tau_phi"
  Gain/1 -> Sum2/2
  omega_psi/1 -> Product/2

== system LQR_2_QuadrotorModel/Subsystem/InverseVirtualControl/Subsystem3 ==
  nu_psi : Inport
  omega_phi : Inport  Port=2
  omega_theta : Inport  Port=3
  coeff : Inport  Port=4
  Gain : Gain  Gain=Ix-Iy
  Gain1 : Gain  Gain=Iz
  Product : Product  Inputs=3
  Sum2 : Sum  Inputs=+-
  tau_psi : Outport
  wires:
  omega_phi/1 -> Product/1
  Gain1/1 -> Sum2/1
  nu_psi/1 -> Gain1/1
  coeff/1 -> Product/3
  Product/1 -> Gain/1
  Sum2/1 -> tau_psi/1  "tau_psi"
  Gain/1 -> Sum2/2
  omega_theta/1 -> Product/2

== system LQR_2_QuadrotorModel/Subsystem/InverseVirtualControl/Subsystem4 ==
  nu_theta : Inport
  omega_phi : Inport  Port=2
  omega_psi : Inport  Port=3
  coeff : Inport  Port=4
  Gain : Gain  Gain=Iz-Ix
  Gain1 : Gain  Gain=Iy
  Product : Product  Inputs=3
  Sum2 : Sum  Inputs=+-
  tau_theta : Outport
  wires:
  omega_phi/1 -> Product/1
  Gain1/1 -> Sum2/1
  nu_theta/1 -> Gain1/1
  coeff/1 -> Product/3
  Product/1 -> Gain/1
  Sum2/1 -> tau_theta/1  "tau_theta"
  Gain/1 -> Sum2/2
  omega_psi/1 -> Product/2

== system LQR_2_QuadrotorModel/Quadrotor/linear motion/Subsystem1/Subsystem2 ==
  T : Inport
  phi : Inport  Port=2
  theta : Inport  Port=3
  psi : Inport  Port=4
  dot_r : Inport  Port=5
  Demux : Demux  Outputs=3
  Subsystem1 : Subsystem
  (F_ind+F_flap)_x : Outport
  (F_ind+F_flap)_y : Outport  Port=2
  (F_ind+F_flap)_z : Outport  Port=3
  wires:
  T/1 -> Subsystem1/5(T)
  Subsystem1/1(F_ind+F_flap) -> Demux/1
  psi/1 -> Subsystem1/3(psi)
  Demux/2 -> (F_ind+F_flap)_y/1  "(F_ind+F_flap)_y"
  dot_r/1 -> Subsystem1/4(dot_r)
  theta/1 -> Subsystem1/2(theta)
  phi/1 -> Subsystem1/1(phi)
  Demux/1 -> (F_ind+F_flap)_x/1  "(F_ind+F_flap)_x"
  Demux/3 -> (F_ind+F_flap)_z/1  "(F_ind+F_flap)_z"

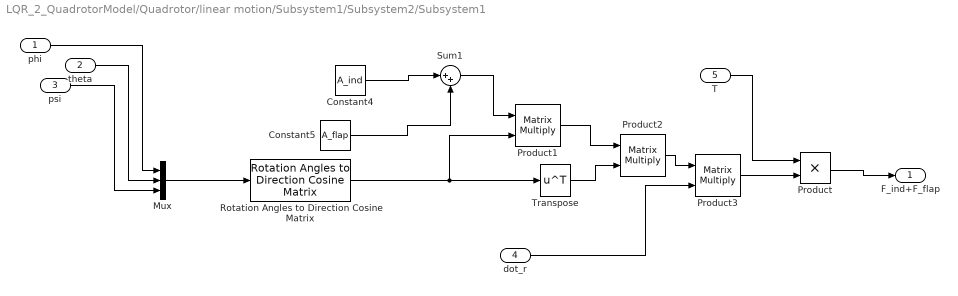
== system LQR_2_QuadrotorModel/Quadrotor/linear motion/Subsystem1/Subsystem2/Subsystem1 ==
  phi : Inport
  theta : Inport  Port=2
  psi : Inport  Port=3
  dot_r : Inport  Port=4
  T : Inport  Port=5
  Constant4 : Constant  Value=A_ind
  Constant5 : Constant  Value=A_flap
  Mux : Mux  Inputs=3
  Product : Product
  Product1 : Product  Multiplication=Matrix(*)
  Product2 : Product  Multiplication=Matrix(*)
  Product3 : Product  Multiplication=Matrix(*)
  Rotation Angles to Direction Cosine Matrix : sharedtransform/Rotation Angles to Direction Cosine Matrix  rotationOrder=ZYX  aMode=aMode
  Sum1 : Sum  Inputs=|++
  Transpose : Math  Operator=transpose
  F_ind+F_flap : Outport
  wires:
  Constant4/1 -> Sum1/1
  Product1/1 -> Product2/1
  Sum1/1 -> Product1/1
  Constant5/1 -> Sum1/2
  psi/1 -> Mux/3
  Product2/1 -> Product3/1
  Rotation Angles to Direction Cosine Matrix/1 -> Product1/2, Transpose/1
  theta/1 -> Mux/2
  Mux/1 -> Rotation Angles to Direction Cosine Matrix/1
  Transpose/1 -> Product2/2
  phi/1 -> Mux/1
  dot_r/1 -> Product3/2
  Product3/1 -> Product/2
  Product/1 -> F_ind+F_flap/1
  T/1 -> Product/1

== matlab function LQR_2_QuadrotorModel/Target Trajectory/MATLAB Function1 ==
  data: t input; x_ref output
function x_ref = trajectory(t)
%#codegen

% Параметры восьмерки
A = 10;      % амплитуда по x
B = 6.5;    % амплитуда по y
h = 5;      % высота
w = 0.2;    % частота

% Параметризация
x = A * sin(w * t);
y = B * sin(w * t) * cos(w * t);
z = h;

% Вычислим производные для курса
dx = A * w * cos(w * t);
dy = B * w * cos(2 * w * t);

% Курс (ориентация по траектории)
psi = atan2(dy, dx);  % направление движенияs

% Выход
x_ref = [x; y; z; 0;0;0;0;0; psi;0;0;0];
end

== matlab function LQR_2_QuadrotorModel/Subsystem/MATLAB Function3 ==
  data: tilde_phi input; tilde_theta input; tilde_omega_phi input; tilde_omega_theta input; nu_phi output; K input; nu_theta output
function [nu_phi, nu_theta]= fcn(tilde_phi, tilde_theta,tilde_omega_phi,tilde_omega_theta, K)

nu_phi = -K(4,1)*tilde_phi-K(4,2)*tilde_omega_phi;
nu_theta = -K(5,1)*tilde_theta-K(5,2)*tilde_omega_theta;

== matlab function LQR_2_QuadrotorModel/Target Trajectory/MATLAB Function ==
  data: t input; forward_20 input; x_ref output; forward_10 input; up_down input; total_time input
function x_ref = trajectory(t, forward_20, forward_10, up_down, total_time)
    % Доля времени на повороты
    turn_time_ratio = 0.2;
    total_turn_time = total_time * turn_time_ratio;
    total_linear_time = total_time - total_turn_time;

    % Время на каждый поворот
    turn_time = total_turn_time / 4;

    % Линейные сегменты разбиты на движение по XY и по Z (всего 8 отрезков)
    % Формат: [dx, dy, dz, dpsi]
    segments = [
        forward_20, 0, 0, 0;       % вперед
        0, 0, up_down, 0;          % вверх
        0, 0, 0, -pi/2;             % поворот влево
        forward_10, 0, 0, 0;       % вперед
        0, 0, -up_down, 0;         % вниз
        0, 0, 0, -pi/2;             % поворот влево
        forward_20, 0, 0, 0;       % вперед
        0, 0, up_down, 0;          % вверх
        0, 0, 0, -pi/2;             % поворот влево
        forward_10, 0, 0, 0;       % вперед
        0, 0, -up_down, 0;         % вниз
        0, 0, 0, -pi/2;             % поворот влево
    ];

    % Определяем длину каждого линейного сегмента
    segment_lengths = vecnorm(segments(:, 1:3), 2, 2);
    total_path_length = sum(segment_lengths);
    
    % Распределяем время на каждый линейный сегмент пропорционально длине
    segment_times = zeros(size(segments, 1), 1);
    for i = 1:size(segments, 1)
        if segments(i, 4) == 0 % линейное движение
            segment_times(i) = segment_lengths(i) / total_path_length * total_linear_time;
        else % поворот
            segment_times(i) = turn_time;
        end
    end

    % Инициализация
    current_x = 0;
    current_y = 0;
    current_z = 0;
    current_psi = 0;
    accumulated_time = 0;

    % Обход сегментов
    for s = 1:size(segments, 1)
        dt = segment_times(s);
        if t <= accumulated_time + dt || s == size(segments,1)
            % Текущий сегмент
            segment_progress = (t - accumulated_time) / dt;
            segment_progress = max(0, min(1, segment_progress));

            dx = segments(s, 1) * segment_progress;
            dy = segments(s, 2) * segment_progress;
            dz = segments(s, 3) * segment_progress;
            dpsi = segments(s, 4) * segment_progress;

            % Преобразование координат с учетом текущего поворота
            if dx ~= 0 || dy ~= 0
                R = [cos(current_psi), -sin(current_psi);
                     sin(current_psi),  cos(current_psi)];
                xy = R * [dx; dy];
            else
                xy = [0; 0];
            end

            x = current_x + xy(1);
            y = current_y + xy(2);
            z = current_z + dz;
            psi = current_psi + dpsi;

            x_ref = [x; y; z; 0; 0; 0; 0; 0; psi; 0; 0; 0];
            return;
        end

        % Завершённый сегмент — обновляем позицию
        dx = segments(s, 1);
        dy = segments(s, 2);
        dz = segments(s, 3);
        dpsi = segments(s, 4);

        if dx ~= 0 || dy ~= 0
            R = [cos(current_psi), -sin(current_psi);
                 sin(current_psi),  cos(current_psi)];
            xy = R * [dx; dy];
        else
            xy = [0; 0];
        end

        current_x = current_x + xy(1);
        current_y = current_y + xy(2);
        current_z = current_z + dz;
        current_psi = current_psi + dpsi;

        accumulated_time = accumulated_time + segment_times(s);
    end

    % Если всё завершено — остаёмся в конечной точке
    x_ref = [current_x; current_y; current_z; 0; 0; 0; 0; 0; current_psi; 0; 0; 0];
end

== matlab function LQR_2_QuadrotorModel/Subsystem/MATLAB Function4 ==
  data: bar_x input; nu output; K input
function nu = fcn(bar_x, K)

nu_x = -K(1,1)*bar_x(1)-K(1,2)*bar_x(4);
nu_y = -K(2,1)*bar_x(2)-K(2,2)*bar_x(5);
nu_z = -K(3,1)*bar_x(3)-K(3,2)*bar_x(6);
nu_psi = -K(6,1)*bar_x(9)-K(6,2)*bar_x(12);


nu = [nu_x; nu_y; nu_z; nu_psi];
